simulink model "v_3_MFCm_load"  (R2023b)
settings: Solver=VariableStepAuto  StartTime=0.0  StopTime=17.0  RelTol=1e-3
values from neighbouring files (symbols this model uses):
  L1 = 0.3    [params.mat]    (also in to_be_opened_before_starting_script.mat)
  L2loaded = 0.25    [params.mat]    (also in to_be_opened_before_starting_script.mat)
  m1 = 4    [params.mat]    (also in to_be_opened_before_starting_script.mat)
  m2loaded = 4    [params.mat]    (also in to_be_opened_before_starting_script.mat)
  x1 = [10.0802901696 16.8958282446 6.48772839028]    [to_be_opened_before_starting_script.mat]
undefined symbols (not defined in the file or in its folder): DiscIntNeverNeededParam, pid_v_MFCm_load
libraries: slpidlib x2, simulink x1
settings Model: Creator=Jan Wyrwicz  LastModifiedBy=Jan Wyrwicz

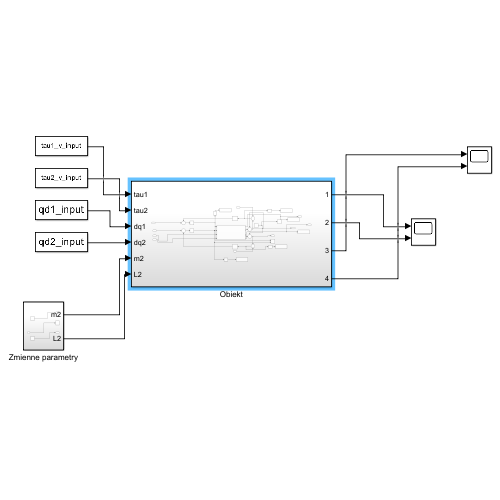
[thumbnail: Simulink's stored preview of the top-level diagram]
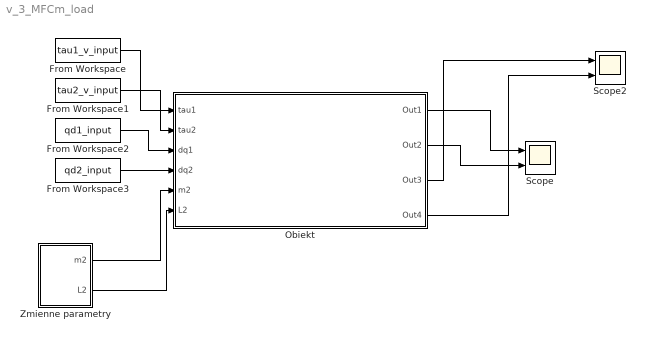
== system v_3_MFCm_load ==
  From Workspace : FromWorkspace  VariableName=tau1_v_input
  From Workspace1 : FromWorkspace  VariableName=tau2_v_input
  From Workspace2 : FromWorkspace  VariableName=qd1_input
  From Workspace3 : FromWorkspace  VariableName=qd2_input
  Obiekt : Subsystem
  Scope : Scope  NumInputPorts=2
  Scope2 : Scope  NumInputPorts=2
  Zmienne parametry : Subsystem
  wires:
  Zmienne parametry/2(L2) -> Obiekt/6(L2)
  Obiekt/2(Out2) -> Scope/2
  Obiekt/1(Out1) -> Scope/1
  Obiekt/3(Out3) -> Scope2/1
  Zmienne parametry/1(m2) -> Obiekt/5(m2)
  Obiekt/4(Out4) -> Scope2/2
  From Workspace3/1 -> Obiekt/4(dq2)
  From Workspace2/1 -> Obiekt/3(dq1)
  From Workspace1/1 -> Obiekt/2(tau2)
  From Workspace/1 -> Obiekt/1(tau1)

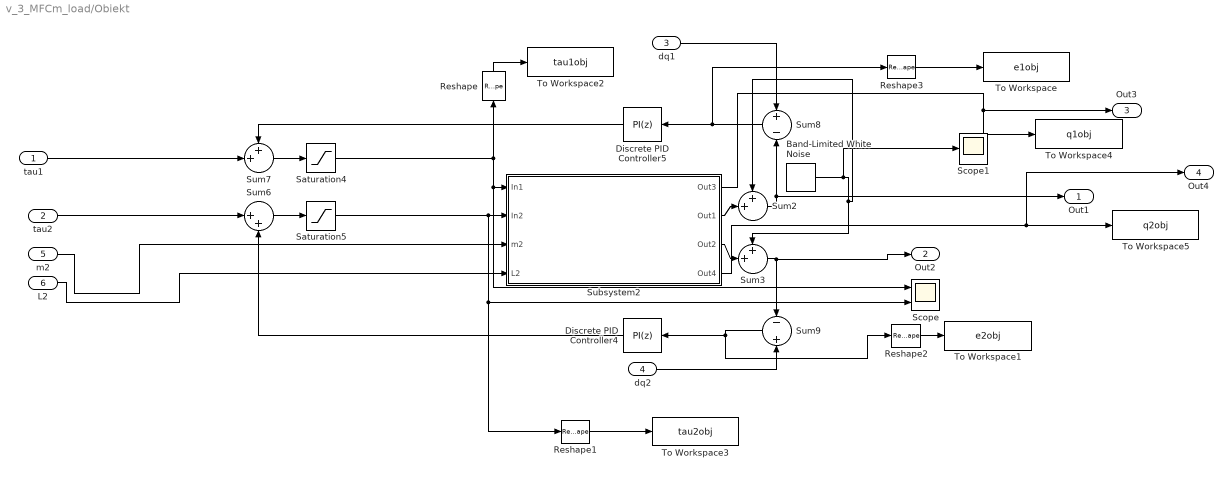
== system v_3_MFCm_load/Obiekt ==
  tau1 : Inport
  tau2 : Inport  Port=2
  dq1 : Inport  Port=3
  dq2 : Inport  Port=4
  m2 : Inport  Port=5
  L2 : Inport  Port=6
  Band-Limited White Noise : simulink/Sources/Band-Limited White Noise  Cov=[0.00000]  Ts=0.001  seed=[23341]
  Discrete PID Controller4 : slpidlib/PID Controller  Controller=PI  Form=Parallel  TimeDomain=Discrete-time  UseExternalTs=off  SampleTime=-1  IntegratorMethod=Forward Euler  FilterMethod=Forward Euler  ControllerParametersSource=internal  P=pid_v_MFCm_load(15,3)  I=pid_v_MFCm_load(15,4)  UseKiTs=off  D=0  N=1000  UseFilter=on  TunerSelectOption=Transfer Function Based (PID Tuner App)  InitialConditionSource=internal  InitialConditionForIntegrator=0  InitialConditionForFilter=0  DifferentiatorICPrevScaledInput=0  ExternalReset=none  TrackingMode=off  Kt=1  LimitOutput=off  SatLimitsSource=internal  UpperSaturationLimit=inf  LowerSaturationLimit=-inf  LinearizeAsGain=off  AntiWindupMode=none  Kb=1  LimitIntegrator=off  UpperIntegratorSaturationLimit=inf  LowerIntegratorSaturationLimit=-inf  POutMin=[]  POutMax=[]  IOutMin=[]  IOutMax=[]  DOutMin=[]  DOutMax=[]  NOutMin=[]  NOutMax=[]  SumOutMin=[]  SumOutMax=[]  SaturationOutMin=[]  SaturationOutMax=[]  PParamMin=[]  PParamMax=[]  IParamMin=[]  IParamMax=[]  DParamMin=[]  DParamMax=[]  NParamMin=[]  NParamMax=[]  KbParamMin=[]  KbParamMax=[]  KtParamMin=[]  KtParamMax=[]  KbOutMin=[]  KbOutMax=[]  KtOutMin=[]  KtOutMax=[]  IntegratorOutMin=[]  IntegratorOutMax=[]  FilterOutMin=[]  FilterOutMax=[]  SumI1OutMin=[]  SumI1OutMax=[]  SumI2OutMin=[]  SumI2OutMax=[]  SumI3OutMin=[]  SumI3OutMax=[]  SumI4OutMin=[]  SumI4OutMax=[]  SumDOutMin=[]  SumDOutMax=[]  DifferentiatorOutMin=[]  DifferentiatorOutMax=[]  FilterDiffOutCoefMin=[]  FilterDiffOutCoefMax=[]  ReciprocalOutMin=[]  ReciprocalOutMax=[]  SumDenOutMin=[]  SumDenOutMax=[]  SumNumOutMin=[]  SumNumOutMax=[]  DivideOutMin=[]  DivideOutMax=[]  UdiffTsProdOutMin=[]  UdiffTsProdOutMax=[]  NTsProdOutMin=[]  NTsProdOutMax=[]  UintegralTsProdOutMin=[]  UintegralTsProdOutMax=[]  UngainTsProdOutMin=[]  UngainTsProdOutMax=[]  ClampingZeroOutDataTypeStr=Inherit: Inherit via back propagation  ClampingZeroOutMin=[]  ClampingZeroOutMax=[]  FilterDenConstantOutDataTypeStr=Inherit: Inherit via back propagation  FilterDenConstantOutMin=[]  FilterDenConstantOutMax=[]  PCopyOutDataTypeStr=Inherit: Inherit via back propagation  PCopyOutMin=[]  PCopyOutMax=[]  NCopyOutDataTypeStr=Inherit: Inherit via back propagation  NCopyOutMin=[]  NCopyOutMax=[]  IntegratorContinuousStateAttributes=''  IntegratorStateMustResolveToSignalObject=off  IntegratorRTWStateStorageClass=Auto  FilterContinuousStateAttributes=''  FilterStateMustResolveToSignalObject=off  FilterRTWStateStorageClass=Auto  ParallelPVariant=InternalParameters  IdealPVariant=Disabled  IVariant=InternalParameters  DVariant=Disabled  IntegratorVariant=Discrete  SatVariant=Disabled  AWVariant=Passthrough  PCopyVariant=Disabled  TRVariant=Disabled  FdbkBlocksVariant=Forward  IdealPFdbkVariant=Disabled  SatFdbkVariant=Disabled  DerivativeFilterVariant=Disabled  NVariant=Disabled  NCopyVariant=Disabled_SignalSpec  FilterICVariant=Disabled  IntegratorICVariant=InternalICs  ExternalResetVariant=Disabled  TRSumVariant=Passthrough  SumFdbkVariant=Disabled  SumVariant=Sum_PI  TsampFilterVariant=InternalTs  TsampNgainVariant=Passthrough  TsampIntegralVariant=Disabled_SignalSpec  ExternalSaturationOutDataTypeStr=Inherit: Same as second input
      settings: LibrarySourceBlock=hdlsllib/Discrete/Discrete PID Controller
  Discrete PID Controller5 : slpidlib/PID Controller  Controller=PI  Form=Parallel  TimeDomain=Discrete-time  UseExternalTs=off  SampleTime=-1  IntegratorMethod=Forward Euler  FilterMethod=Forward Euler  ControllerParametersSource=internal  P=pid_v_MFCm_load(15,1)  I=pid_v_MFCm_load(15,2)  UseKiTs=off  D=x1(3)  N=1000  UseFilter=on  TunerSelectOption=Transfer Function Based (PID Tuner App)  InitialConditionSource=internal  InitialConditionForIntegrator=0  InitialConditionForFilter=0  DifferentiatorICPrevScaledInput=0  ExternalReset=none  TrackingMode=off  Kt=1  LimitOutput=off  SatLimitsSource=internal  UpperSaturationLimit=inf  LowerSaturationLimit=-inf  LinearizeAsGain=off  AntiWindupMode=none  Kb=1  LimitIntegrator=off  UpperIntegratorSaturationLimit=inf  LowerIntegratorSaturationLimit=-inf  POutMin=[]  POutMax=[]  IOutMin=[]  IOutMax=[]  DOutMin=[]  DOutMax=[]  NOutMin=[]  NOutMax=[]  SumOutMin=[]  SumOutMax=[]  SaturationOutMin=[]  SaturationOutMax=[]  PParamMin=[]  PParamMax=[]  IParamMin=[]  IParamMax=[]  DParamMin=[]  DParamMax=[]  NParamMin=[]  NParamMax=[]  KbParamMin=[]  KbParamMax=[]  KtParamMin=[]  KtParamMax=[]  KbOutMin=[]  KbOutMax=[]  KtOutMin=[]  KtOutMax=[]  IntegratorOutMin=[]  IntegratorOutMax=[]  FilterOutMin=[]  FilterOutMax=[]  SumI1OutMin=[]  SumI1OutMax=[]  SumI2OutMin=[]  SumI2OutMax=[]  SumI3OutMin=[]  SumI3OutMax=[]  SumI4OutMin=[]  SumI4OutMax=[]  SumDOutMin=[]  SumDOutMax=[]  DifferentiatorOutMin=[]  DifferentiatorOutMax=[]  FilterDiffOutCoefMin=[]  FilterDiffOutCoefMax=[]  ReciprocalOutMin=[]  ReciprocalOutMax=[]  SumDenOutMin=[]  SumDenOutMax=[]  SumNumOutMin=[]  SumNumOutMax=[]  DivideOutMin=[]  DivideOutMax=[]  UdiffTsProdOutMin=[]  UdiffTsProdOutMax=[]  NTsProdOutMin=[]  NTsProdOutMax=[]  UintegralTsProdOutMin=[]  UintegralTsProdOutMax=[]  UngainTsProdOutMin=[]  UngainTsProdOutMax=[]  ClampingZeroOutDataTypeStr=Inherit: Inherit via back propagation  ClampingZeroOutMin=[]  ClampingZeroOutMax=[]  FilterDenConstantOutDataTypeStr=Inherit: Inherit via back propagation  FilterDenConstantOutMin=[]  FilterDenConstantOutMax=[]  PCopyOutDataTypeStr=Inherit: Inherit via back propagation  PCopyOutMin=[]  PCopyOutMax=[]  NCopyOutDataTypeStr=Inherit: Inherit via back propagation  NCopyOutMin=[]  NCopyOutMax=[]  IntegratorContinuousStateAttributes=''  IntegratorStateMustResolveToSignalObject=off  IntegratorRTWStateStorageClass=Auto  FilterContinuousStateAttributes=''  FilterStateMustResolveToSignalObject=off  FilterRTWStateStorageClass=Auto  ParallelPVariant=InternalParameters  IdealPVariant=Disabled  IVariant=InternalParameters  DVariant=Disabled  IntegratorVariant=Discrete  SatVariant=Disabled  AWVariant=Passthrough  PCopyVariant=Disabled  TRVariant=Disabled  FdbkBlocksVariant=Forward  IdealPFdbkVariant=Disabled  SatFdbkVariant=Disabled  DerivativeFilterVariant=Disabled  NVariant=Disabled  NCopyVariant=Disabled_SignalSpec  FilterICVariant=Disabled  IntegratorICVariant=InternalICs  ExternalResetVariant=Disabled  TRSumVariant=Passthrough  SumFdbkVariant=Disabled  SumVariant=Sum_PI  TsampFilterVariant=InternalTs  TsampNgainVariant=Passthrough  TsampIntegralVariant=Disabled_SignalSpec  ExternalSaturationOutDataTypeStr=Inherit: Same as second input
      settings: LibrarySourceBlock=hdlsllib/Discrete/Discrete PID Controller
  Reshape{,1..3} (4 alike) : Reshape
  Saturation4 : Saturate  UpperLimit=40  LowerLimit=-40
  Saturation5 : Saturate  UpperLimit=15  LowerLimit=-15
  Scope : Scope  NumInputPorts=2
  Scope1 : Scope
  Subsystem2 : Subsystem
  Sum2 : Sum  Inputs=++|
  Sum3 : Sum  Inputs=++|
  Sum6 : Sum  Inputs=|++
  Sum7 : Sum  Inputs=++|
  Sum8 : Sum  Inputs=+|-
  Sum9 : Sum  Inputs=-|+
  To Workspace : ToWorkspace  VariableName=e1obj  SampleTime=-1
      settings: Save2DSignal=2-D array (concatenate along first dimension)
  To Workspace1 : ToWorkspace  VariableName=e2obj  SampleTime=-1
      settings: Save2DSignal=2-D array (concatenate along first dimension)
  To Workspace2 : ToWorkspace  VariableName=tau1obj  SampleTime=-1
      settings: Save2DSignal=2-D array (concatenate along first dimension)
  To Workspace3 : ToWorkspace  VariableName=tau2obj  SampleTime=-1
      settings: Save2DSignal=2-D array (concatenate along first dimension)
  To Workspace4 : ToWorkspace  VariableName=q1obj  SampleTime=-1
      settings: Save2DSignal=2-D array (concatenate along first dimension)
  To Workspace5 : ToWorkspace  VariableName=q2obj  SampleTime=-1
      settings: Save2DSignal=2-D array (concatenate along first dimension)
  Out1 : Outport
  Out2 : Outport  Port=2
  Out3 : Outport  Port=3
  Out4 : Outport  Port=4
  wires:
  tau2/1 -> Sum6/1
  Sum6/1 -> Saturation5/1
  tau1/1 -> Sum7/2
  Sum7/1 -> Saturation4/1
  Saturation4/1 -> Scope/1, Subsystem2/1(In1), Reshape/1
  Saturation5/1 -> Scope/2, Reshape1/1, Subsystem2/2(In2)
  Sum9/1 -> Reshape2/1, Discrete PID Controller4/1
  Discrete PID Controller4/1 -> Sum6/2
  Sum8/1 -> Reshape3/1, Discrete PID Controller5/1
  Discrete PID Controller5/1 -> Sum7/1
  dq1/1 -> Sum8/1
  dq2/1 -> Sum9/2
  m2/1 -> Subsystem2/3(m2)
  L2/1 -> Subsystem2/4(L2)
  Band-Limited White Noise/1 -> Scope1/1, Sum3/1, Sum2/1
  Subsystem2/3(Out2) -> Sum3/2
  Subsystem2/2(Out1) -> Sum2/2
  Sum2/1 -> Out1/1, Sum8/2
  Subsystem2/1(Out3) -> To Workspace4/1, Out3/1
  Subsystem2/4(Out4) -> Out4/1, To Workspace5/1
  Sum3/1 -> Sum9/1, Out2/1
  Reshape/1 -> To Workspace2/1
  Reshape1/1 -> To Workspace3/1
  Reshape2/1 -> To Workspace1/1
  Reshape3/1 -> To Workspace/1

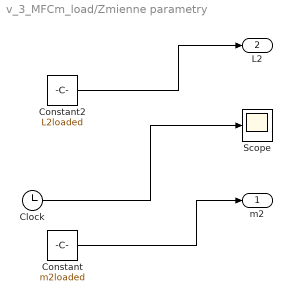
== system v_3_MFCm_load/Zmienne parametry ==
  Clock : Clock
  Constant : Constant  Value=m2loaded
  Constant2 : Constant  Value=L2loaded
  Scope : Scope
  m2 : Outport
  L2 : Outport  Port=2
  wires:
  Constant/1 -> m2/1
  Clock/1 -> Scope/1
  Constant2/1 -> L2/1

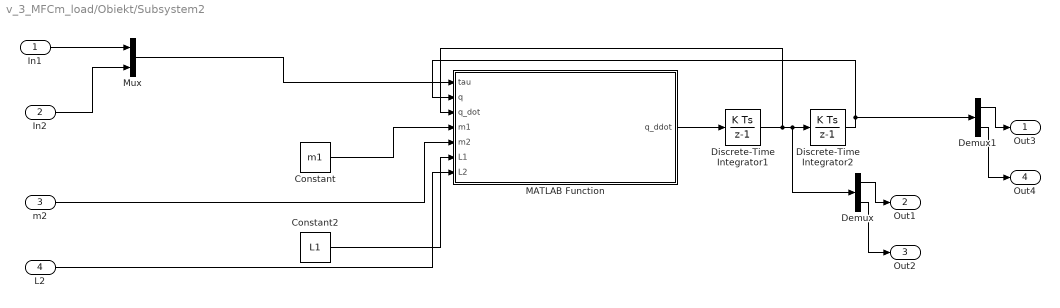
== system v_3_MFCm_load/Obiekt/Subsystem2 ==
  In1 : Inport
  In2 : Inport  Port=2
  m2 : Inport  Port=3
  L2 : Inport  Port=4
  Constant : Constant  Value=m1
  Constant2 : Constant  Value=L1
  Demux : Demux  Outputs=2
  Demux1 : Demux  Outputs=2
  Discrete-Time Integrator1 : DiscreteIntegrator  SampleTime=-1  ICPrevOutput=DiscIntNeverNeededParam  ICPrevScaledInput=DiscIntNeverNeededParam
  Discrete-Time Integrator2 : DiscreteIntegrator  SampleTime=-1  ICPrevOutput=DiscIntNeverNeededParam  ICPrevScaledInput=DiscIntNeverNeededParam
  MATLAB Function : MATLAB Function  TreatAsAtomicUnit=on
  Mux : Mux  Inputs=2
  Out3 : Outport
  Out1 : Outport  Port=2
  Out2 : Outport  Port=3
  Out4 : Outport  Port=4
  wires:
  MATLAB Function/1(q_ddot) -> Discrete-Time Integrator1/1
  Discrete-Time Integrator1/1 -> Demux/1, Discrete-Time Integrator2/1, MATLAB Function/3(q_dot)
  Mux/1 -> MATLAB Function/1(tau)
  Constant/1 -> MATLAB Function/4(m1)
  m2/1 -> MATLAB Function/5(m2)
  Constant2/1 -> MATLAB Function/6(L1)
  L2/1 -> MATLAB Function/7(L2)
  Demux/1 -> Out1/1
  Demux/2 -> Out2/1
  In1/1 -> Mux/1
  In2/1 -> Mux/2
  Discrete-Time Integrator2/1 -> Demux1/1, MATLAB Function/2(q)
  Demux1/2 -> Out4/1
  Demux1/1 -> Out3/1

== matlab function v_3_MFCm_load/Obiekt/Subsystem2/MATLAB Function ==
  data: tau input; q_ddot output size=[2,1]; q input; q_dot input; m1 input; m2 input; L1 input; L2 input
function q_ddot  = inverse_dynamics(tau,q,q_dot,m1,m2,L1,L2)

g = 9.8067;

invM = [                          1/(L1^2*m1 + L1^2*m2 - L1^2*m2*cos(q(2))^2),                                                -(L2 + L1*cos(q(2)))/(L1^2*L2*m1 + L1^2*L2*m2 - L1^2*L2*m2*cos(q(2))^2);...
        -(L2 + L1*cos(q(2)))/(L1^2*L2*m1 + L1^2*L2*m2 - L1^2*L2*m2*cos(q(2))^2), (L1^2*m1 + L1^2*m2 + L2^2*m2 + 2*L1*L2*m2*cos(q(2)))/(- L1^2*L2^2*m2^2*cos(q(2))^2 + L1^2*L2^2*m2^2 + m1*L1^2*L2^2*m2)];


c = [-m2*L1*L2*sin(q(2))*(2*q_dot(1)*q_dot(2) + q_dot(2)^2); m2*L1*L2*q_dot(1)^2*sin(q(2))];

G = [(m1 + m2)*L1*g*cos(q(1)) + m2*g*L2*cos(q(1) + q(2));  m2*g*L2*cos(q(1) + q(2))];


q_ddot = invM*(tau - c - G);
